simulink model "motorcycle_kinematics_observer"  (R2022b)
settings: Solver=VariableStepAuto  StartTime=0.0  StopTime=tf  MaxStep=ts  RelTol=1e-3
InitFcn:
  | motorcycle_kinematics_observer_init;
values from neighbouring files (symbols this model uses):
  params = [ ... (first row only)    [motorcycle_kinematics_observer_init.m]
  q0 = q.Data(1,:)    [motorcycle_kinematics_observer_init.m]
settings Model: Creator=marti  LastModifiedBy=marti

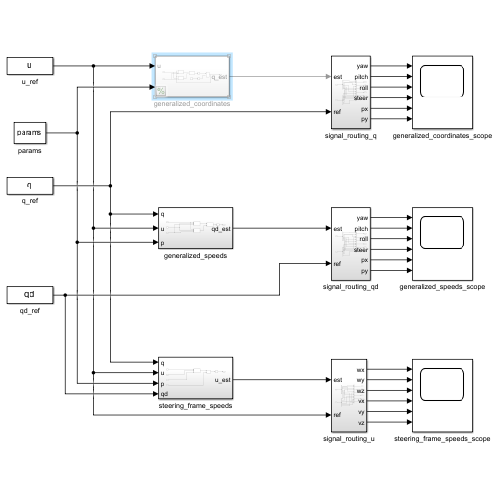
[thumbnail: Simulink's stored preview of the top-level diagram]
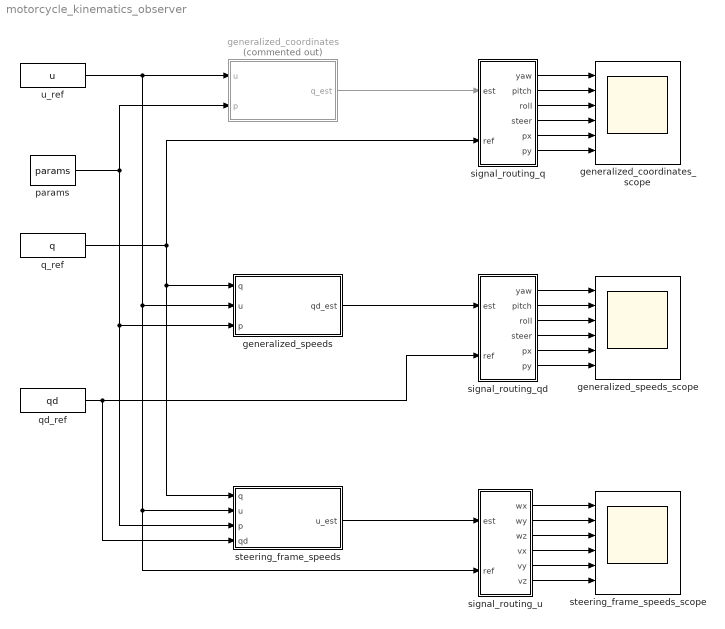
== system motorcycle_kinematics_observer ==
  generalized_coordinates : Subsystem  Commented=on
  generalized_coordinates_scope : Scope  NumInputPorts=6
  generalized_speeds : Subsystem
  generalized_speeds_scope : Scope  NumInputPorts=6
  params : Constant  Value=params
  q_ref : FromWorkspace  VariableName=q
  qd_ref : FromWorkspace  VariableName=qd
  signal_routing_q : Subsystem
  signal_routing_qd : Subsystem
  signal_routing_u : Subsystem
  steering_frame_speeds : Subsystem
  steering_frame_speeds_scope : Scope  NumInputPorts=6
  u_ref : FromWorkspace  VariableName=u
  wires:
  q_ref/1 -> signal_routing_q/2(ref), steering_frame_speeds/1(q), generalized_speeds/1(q)
  signal_routing_q/1(yaw) -> generalized_coordinates_scope/1
  signal_routing_q/2(pitch) -> generalized_coordinates_scope/2
  signal_routing_q/3(roll) -> generalized_coordinates_scope/3
  signal_routing_q/4(steer) -> generalized_coordinates_scope/4
  signal_routing_q/5(px) -> generalized_coordinates_scope/5
  signal_routing_q/6(py) -> generalized_coordinates_scope/6
  u_ref/1 -> generalized_coordinates/1(u), steering_frame_speeds/2(u), signal_routing_u/2(ref), generalized_speeds/2(u)
  params/1 -> generalized_coordinates/2(p), steering_frame_speeds/3(p), generalized_speeds/3(p)
  generalized_coordinates/1(q_est) -> signal_routing_q/1(est)
  qd_ref/1 -> signal_routing_qd/2(ref), steering_frame_speeds/4(qd)
  signal_routing_u/1(wx) -> steering_frame_speeds_scope/1
  signal_routing_u/2(wy) -> steering_frame_speeds_scope/2
  signal_routing_u/3(wz) -> steering_frame_speeds_scope/3
  signal_routing_u/4(vx) -> steering_frame_speeds_scope/4
  signal_routing_u/5(vy) -> steering_frame_speeds_scope/5
  signal_routing_u/6(vz) -> steering_frame_speeds_scope/6
  steering_frame_speeds/1(u_est) -> signal_routing_u/1(est)
  signal_routing_qd/6(py) -> generalized_speeds_scope/6
  signal_routing_qd/5(px) -> generalized_speeds_scope/5
  signal_routing_qd/4(steer) -> generalized_speeds_scope/4
  signal_routing_qd/3(roll) -> generalized_speeds_scope/3
  signal_routing_qd/2(pitch) -> generalized_speeds_scope/2
  signal_routing_qd/1(yaw) -> generalized_speeds_scope/1
  generalized_speeds/1(qd_est) -> signal_routing_qd/1(est)

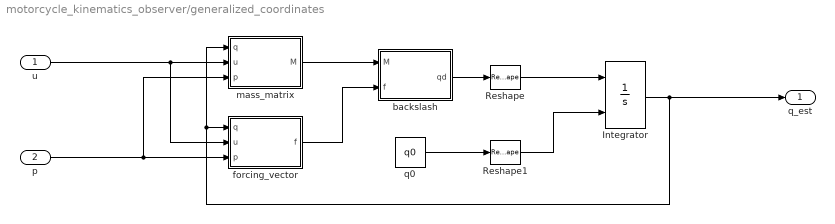
== system motorcycle_kinematics_observer/generalized_coordinates ==
  u : Inport
  p : Inport  Port=2
  Integrator : Integrator  InitialConditionSource=external  WrapState=on  WrappedStateUpperValue=[pi.*ones(1,4),inf(1,2)]  WrappedStateLowerValue=-[pi.*ones(1,4),inf(1,2)]
  Reshape : Reshape
  Reshape1 : Reshape
  backslash : MATLAB Function  TreatAsAtomicUnit=on
  forcing_vector : MATLAB Function  TreatAsAtomicUnit=on
  mass_matrix : MATLAB Function  TreatAsAtomicUnit=on
  q0 : Constant  Value=q0
  q_est : Outport
  wires:
  p/1 -> mass_matrix/3(p), forcing_vector/3(p)
  forcing_vector/1(f) -> backslash/2(f)
  Reshape/1 -> Integrator/1
  q0/1 -> Reshape1/1
  Integrator/1 -> q_est/1, mass_matrix/1(q), forcing_vector/1(q)
  u/1 -> forcing_vector/2(u), mass_matrix/2(u)
  backslash/1(qd) -> Reshape/1
  mass_matrix/1(M) -> backslash/1(M)
  Reshape1/1 -> Integrator/2

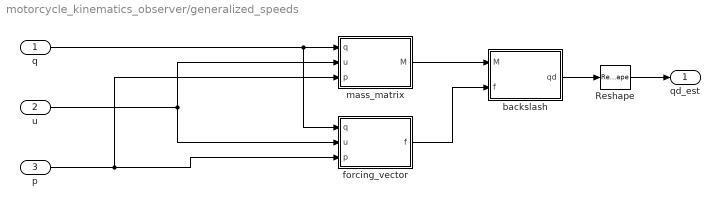
== system motorcycle_kinematics_observer/generalized_speeds ==
  q : Inport
  u : Inport  Port=2
  p : Inport  Port=3
  Reshape : Reshape
  backslash : MATLAB Function  TreatAsAtomicUnit=on
  forcing_vector : MATLAB Function  TreatAsAtomicUnit=on
  mass_matrix : MATLAB Function  TreatAsAtomicUnit=on
  qd_est : Outport
  wires:
  forcing_vector/1(f) -> backslash/2(f)
  Reshape/1 -> qd_est/1
  backslash/1(qd) -> Reshape/1
  mass_matrix/1(M) -> backslash/1(M)
  q/1 -> forcing_vector/1(q), mass_matrix/1(q)
  u/1 -> forcing_vector/2(u), mass_matrix/2(u)
  p/1 -> forcing_vector/3(p), mass_matrix/3(p)

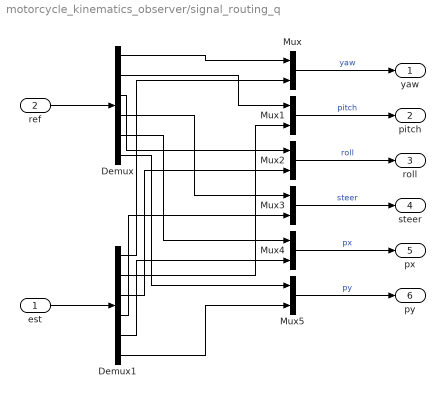
== system motorcycle_kinematics_observer/signal_routing_q ==
  est : Inport
  ref : Inport  Port=2
  Demux : Demux  Outputs=6
  Demux1 : Demux  Outputs=6
  Mux{,1..5} (6 alike) : Mux  Inputs=2
  yaw : Outport
  pitch : Outport  Port=2
  roll : Outport  Port=3
  steer : Outport  Port=4
  px : Outport  Port=5
  py : Outport  Port=6
  wires:
  Demux/6 -> Mux5/1
  Mux1/1 -> pitch/1  "pitch"
  Demux/2 -> Mux1/1
  Demux/4 -> Mux3/1
  Demux1/4 -> Mux3/2
  Demux/3 -> Mux2/1
  Demux1/2 -> Mux1/2
  Demux/5 -> Mux4/1
  Demux1/6 -> Mux5/2
  Demux1/1 -> Mux/2
  Demux/1 -> Mux/1
  Demux1/3 -> Mux2/2
  Mux5/1 -> py/1  "py"
  Demux1/5 -> Mux4/2
  Mux/1 -> yaw/1  "yaw"
  Mux3/1 -> steer/1  "steer"
  est/1 -> Demux1/1
  ref/1 -> Demux/1
  Mux2/1 -> roll/1  "roll"
  Mux4/1 -> px/1  "px"

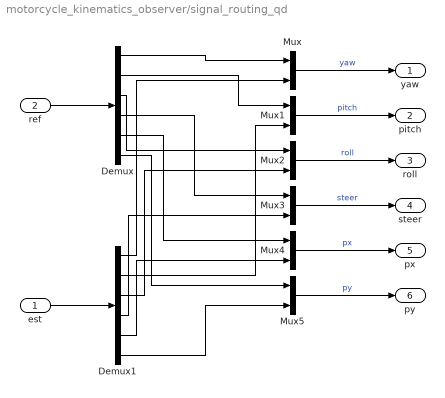
== system motorcycle_kinematics_observer/signal_routing_qd ==
  est : Inport
  ref : Inport  Port=2
  Demux : Demux  Outputs=6
  Demux1 : Demux  Outputs=6
  Mux{,1..5} (6 alike) : Mux  Inputs=2
  yaw : Outport
  pitch : Outport  Port=2
  roll : Outport  Port=3
  steer : Outport  Port=4
  px : Outport  Port=5
  py : Outport  Port=6
  wires:
  Demux/6 -> Mux5/1
  Mux1/1 -> pitch/1  "pitch"
  Demux/2 -> Mux1/1
  Demux/4 -> Mux3/1
  Demux1/4 -> Mux3/2
  Demux/3 -> Mux2/1
  Demux1/2 -> Mux1/2
  Demux/5 -> Mux4/1
  Demux1/6 -> Mux5/2
  Demux1/1 -> Mux/2
  Demux/1 -> Mux/1
  Demux1/3 -> Mux2/2
  Mux5/1 -> py/1  "py"
  Demux1/5 -> Mux4/2
  Mux/1 -> yaw/1  "yaw"
  Mux3/1 -> steer/1  "steer"
  est/1 -> Demux1/1
  ref/1 -> Demux/1
  Mux2/1 -> roll/1  "roll"
  Mux4/1 -> px/1  "px"

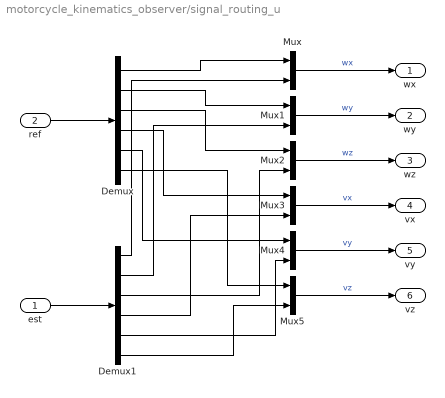
== system motorcycle_kinematics_observer/signal_routing_u ==
  est : Inport
  ref : Inport  Port=2
  Demux : Demux  Outputs=6
  Demux1 : Demux  Outputs=6
  Mux{,1..5} (6 alike) : Mux  Inputs=2
  wx : Outport
  wy : Outport  Port=2
  wz : Outport  Port=3
  vx : Outport  Port=4
  vy : Outport  Port=5
  vz : Outport  Port=6
  wires:
  Mux1/1 -> wy/1  "wy"
  Mux5/1 -> vz/1  "vz"
  Mux/1 -> wx/1  "wx"
  Mux3/1 -> vx/1  "vx"
  est/1 -> Demux1/1
  ref/1 -> Demux/1
  Mux2/1 -> wz/1  "wz"
  Mux4/1 -> vy/1  "vy"
  Demux/1 -> Mux/1
  Demux/2 -> Mux1/1
  Demux/3 -> Mux2/1
  Demux/4 -> Mux3/1
  Demux/5 -> Mux4/1
  Demux/6 -> Mux5/1
  Demux1/1 -> Mux/2
  Demux1/2 -> Mux1/2
  Demux1/3 -> Mux2/2
  Demux1/4 -> Mux3/2
  Demux1/5 -> Mux4/2
  Demux1/6 -> Mux5/2

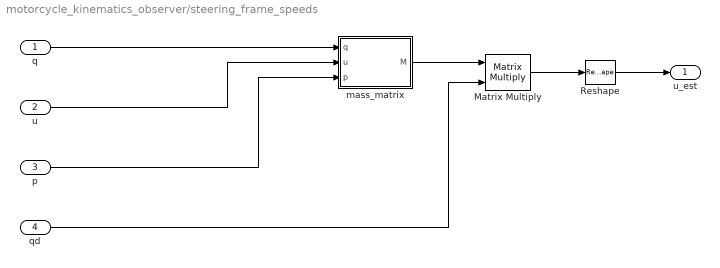
== system motorcycle_kinematics_observer/steering_frame_speeds ==
  q : Inport
  u : Inport  Port=2
  p : Inport  Port=3
  qd : Inport  Port=4
  Matrix Multiply : Product  Multiplication=Matrix(*)
  Reshape : Reshape
  mass_matrix : MATLAB Function  TreatAsAtomicUnit=on
  u_est : Outport
  wires:
  Reshape/1 -> u_est/1
  Matrix Multiply/1 -> Reshape/1
  mass_matrix/1(M) -> Matrix Multiply/1
  q/1 -> mass_matrix/1(q)
  p/1 -> mass_matrix/3(p)
  u/1 -> mass_matrix/2(u)
  qd/1 -> Matrix Multiply/2

== matlab function motorcycle_kinematics_observer/generalized_coordinates/mass_matrix ==
  data: q input; u input; p input; M output
function M = fcn(q,u,p)
M = motorcycleKinematicsMassMatrix(q,u,p);

== matlab function motorcycle_kinematics_observer/generalized_coordinates/backslash ==
  data: M input; qd output; f input
function qd = fcn(M,f)
qd = M\f;

== matlab function motorcycle_kinematics_observer/generalized_speeds/backslash ==
  data: M input; qd output; f input
function qd = fcn(M,f)
qd = M\f;

== matlab function motorcycle_kinematics_observer/generalized_speeds/forcing_vector ==
  data: q input; u input; f output; p input
function f = fcn(q,u,p)
f = motorcycleKinematicsForcingVector(q,u,p);

== matlab function motorcycle_kinematics_observer/generalized_speeds/mass_matrix ==
  data: q input; u input; p input; M output
function M = fcn(q,u,p)
M = motorcycleKinematicsMassMatrix(q,u,p);

== matlab function motorcycle_kinematics_observer/steering_frame_speeds/mass_matrix ==
  data: q input; u input; p input; M output
function M = fcn(q,u,p)
M = motorcycleKinematicsMassMatrix(q,u,p);

== matlab function motorcycle_kinematics_observer/generalized_coordinates/forcing_vector ==
  data: q input; u input; f output; p input
function f = fcn(q,u,p)
f = motorcycleKinematicsForcingVector(q,u,p);
